simulink model "sumOfOddNumbersSimulink"  (R2020b)
settings: Solver=VariableStepAuto  StartTime=0.0  StopTime=10.0  RelTol=1e-3
undefined symbols (not defined in the file or in its folder): n
settings Model: Creator=riwakaram  LastModifiedBy=riwakaram

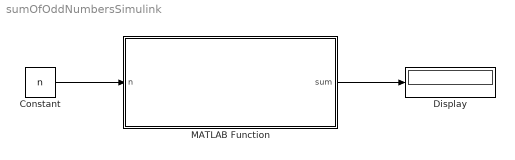
== system sumOfOddNumbersSimulink ==
  Constant : Constant  Value=n
  Display : Display
  MATLAB Function : MATLAB Function  TreatAsAtomicUnit=on
  wires:
  Constant/1 -> MATLAB Function/1(n)
  MATLAB Function/1(sum) -> Display/1

== matlab function sumOfOddNumbersSimulink/MATLAB Function ==
  data: n input; sum output
function sum = sumOfOddNumbers(n)
sum = 0;
    for i = 1:n
        if (mod(i,2) ~= 0)
            sum = sum + i;
        end
    end
sum = sumOfOddNumbers(n);
